simulink model "mechatronic_system_ss"  (R2023b)
settings: Solver=ode1  StartTime=0.0  StopTime=inf  FixedStep=time_step  RelTol=1e-3  EnableMultiTasking=on
model workspace (MAT data in the model file):
  A_ss = [0  1  0  0  0  0; 0  -10.6382978723  0  -2.12765957447  0  0; 0  0  0  1  0  0; 0  8.33333333333  -16666.6666667  -184.166666667  166666.666667  0; 0  0  0  0  0  1; 0  0  1000  0  -10000  -1.5]
  B_ss = [0  0  0  0  0  0; 0  1  0  0  0  0; 0  0  0  0  0  0; 0  0  0  0  0  0; 0  0  0  0  0  0; 0  0  0  0  0  1]
  C_ss = [1  0  0  0  0  0; 0  1  0  0  0  0; 0  0  1  0  0  0; 0  0  0  1  0  0; 0  0  0  0  1  0; 0  0  0  0  0  1]
  Cm = 0.1
  D_ss = [0  0  0  0  0  0; 0  0  0  0  0  0; 0  0  0  0  0  0; 0  0  0  0  0  0; 0  0  0  0  0  0; 0  0  0  0  0  0]
  J_shaft = 0.012
  Ja = 0.001
  La = 0.047
  Ra = 0.5
  b_shaft = 2.21
  b_spring = 3
  ba = 0.01
  g = 9.81
  k_spring = 20000
  lower_limit = 0
  m = 2
  r_shaft = 0.1
  time_step = 0.002
  upper_limit = 5
libraries: simulink x1
settings Model: Creator=danie  LastModifiedBy=danie
settings SolverCC: AutoInsertRateTranBlk=on  InsertRTBMode=Always
settings OptimizationCC: DefaultParameterBehavior=Inlined  EnhancedBackFolding=on  PassReuseOutputArgsAs=Individual arguments  ZeroExternalMemoryAtStartup=off  ZeroInternalMemoryAtStartup=off  OptimizeBlockOrder=speed  DifferentSizesBufferReuse=on  OptimizationCustomize=off  EfficientTunableParamExpr=on
settings DebuggingCC: ParameterTunabilityLossMsg=error
settings HardwareCC: ProdBitPerLong=64  ProdHWDeviceType=Intel->x86-64 (Linux 64)
settings SFSimCC: MATLABDynamicMemAlloc=off
settings RTWCC: Description=Embedded Coder  SystemTargetFile=ert.tlc  GenCodeOnly=on  PackageGeneratedCodeAndArtifacts=on  TemplateMakefile=ert_default_tmf
settings CodeAppCC: ForceParamTrailComments=on  IgnoreCustomStorageClasses=off  OperatorAnnotations=on  SimulinkDataObjDesc=on  SFDataObjDesc=on  InsertBlockDesc=on
settings ERTTargetCC: TargetLangStandard=C99 (ISO)  GenerateSampleERTMain=on  SupportContinuousTime=on  InlinedParameterPlacement=NonHierarchical  ERTCustomFileTemplate=example_file_process.tlc

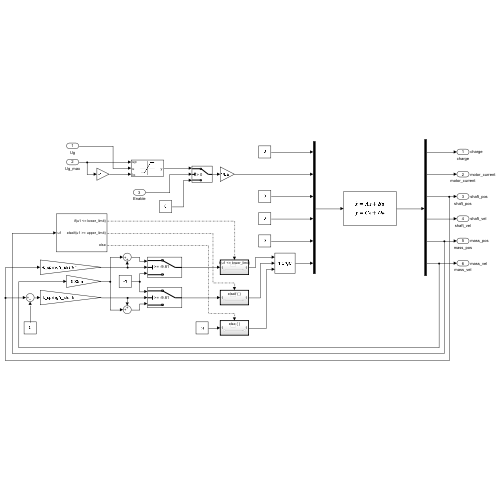
[thumbnail: Simulink's stored preview of the top-level diagram]
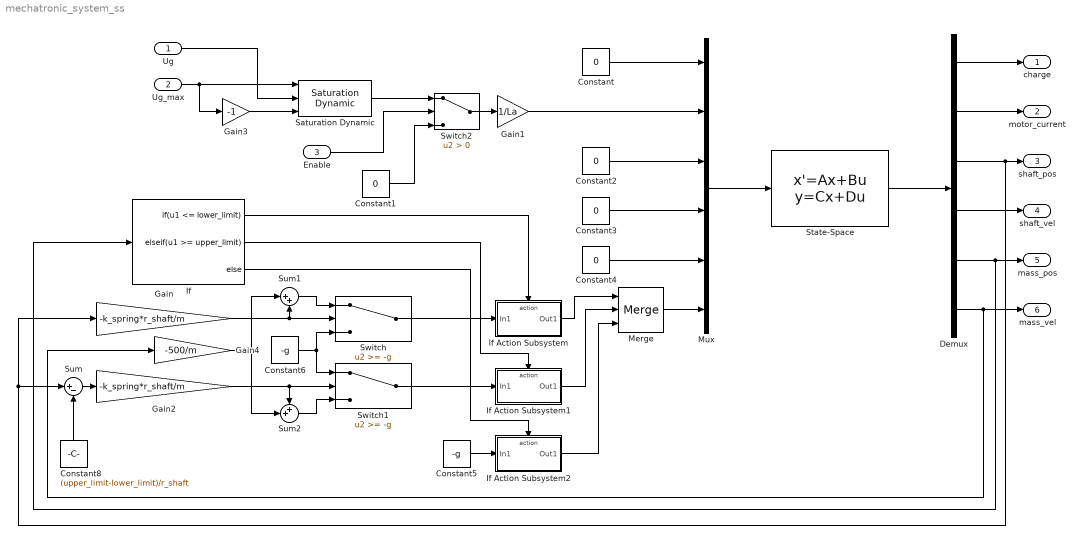
== system mechatronic_system_ss ==
  Ug : Inport
  Ug_max : Inport  Port=2
  Enable : Inport  Port=3
  Constant{,1..4} (5 alike) : Constant  Value=0
  Constant5 : Constant  Value=-g
  Constant6 : Constant  Value=-g
  Constant8 : Constant  Value=(upper_limit-lower_limit)/r_shaft
  Demux : Demux  Outputs=6
  Gain : Gain  Gain=-k_spring*r_shaft/m
  Gain1 : Gain  Gain=1/La
  Gain2 : Gain  Gain=-k_spring*r_shaft/m
  Gain3 : Gain  Gain=-1
  Gain4 : Gain  Gain=-500/m
  If : If  IfExpression=u1 <= lower_limit  ElseIfExpressions=u1 >= upper_limit
  If Action Subsystem : Subsystem  TreatAsAtomicUnit=on
  If Action Subsystem1 : Subsystem  TreatAsAtomicUnit=on
  If Action Subsystem2 : Subsystem  TreatAsAtomicUnit=on
  Merge : Merge  Inputs=3
  Mux : Mux  Inputs=6
  Saturation Dynamic : simulink/Discontinuities/Saturation Dynamic  OutMin=[]  OutMax=[]  OutDataTypeStr=Inherit: Same as second input  OutDataType=fixdt(1, 16)  OutScaling=2^-10  DoSatur=off
  State-Space : StateSpace  A=A_ss  B=B_ss  C=C_ss  D=D_ss  InitialCondition=0
  Sum : Sum  Inputs=|+-
  Sum1 : Sum  Inputs=|++
  Sum2 : Sum  Inputs=++|
  Switch : Switch  Threshold=-g  SaturateOnIntegerOverflow=off  InputSameDT=off
  Switch1 : Switch  Threshold=-g  SaturateOnIntegerOverflow=off  InputSameDT=off
  Switch2 : Switch  Criteria=u2 > Threshold  SaturateOnIntegerOverflow=off  InputSameDT=off
  charge : Outport  SignalName=charge
  motor_current : Outport  Port=2  SignalName=motor_current
  shaft_pos : Outport  Port=3  SignalName=shaft_pos
  shaft_vel : Outport  Port=4  SignalName=shaft_vel
  mass_pos : Outport  Port=5  SignalName=mass_pos
  mass_vel : Outport  Port=6  SignalName=mass_vel
  wires:
  Mux/1 -> State-Space/1
  State-Space/1 -> Demux/1
  Constant/1 -> Mux/1
  Gain1/1 -> Mux/2
  Constant2/1 -> Mux/3
  Constant3/1 -> Mux/4
  Constant4/1 -> Mux/5
  Demux/1 -> charge/1
  Demux/2 -> motor_current/1
  Demux/4 -> shaft_vel/1
  Demux/3 -> shaft_pos/1, Sum/1, Gain/1
  Demux/5 -> mass_pos/1, If/1
  Demux/6 -> Gain4/1, mass_vel/1
  If/1 -> If Action Subsystem/Action
  If/2 -> If Action Subsystem1/Action
  If/3 -> If Action Subsystem2/Action
  Merge/1 -> Mux/6
  If Action Subsystem/1(Out1) -> Merge/1
  If Action Subsystem1/1(Out1) -> Merge/2
  If Action Subsystem2/1(Out1) -> Merge/3
  Switch/1 -> If Action Subsystem/1(In1)
  Switch1/1 -> If Action Subsystem1/1(In1)
  Gain/1 -> Sum1/2, Switch/2
  Constant5/1 -> If Action Subsystem2/1(In1)
  Constant6/1 -> Switch1/1, Switch/3
  Sum/1 -> Gain2/1
  Gain2/1 -> Sum2/1, Switch1/2
  Constant8/1 -> Sum/2
  Gain3/1 -> Saturation Dynamic/3
  Ug/1 -> Saturation Dynamic/2
  Ug_max/1 -> Gain3/1, Saturation Dynamic/1
  Switch2/1 -> Gain1/1
  Saturation Dynamic/1 -> Switch2/1
  Constant1/1 -> Switch2/3
  Enable/1 -> Switch2/2
  Sum1/1 -> Switch/1
  Sum2/1 -> Switch1/3
  Gain4/1 -> Sum1/1, Sum2/2

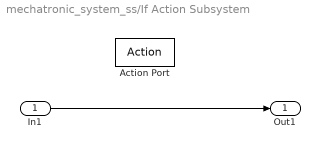
== system mechatronic_system_ss/If Action Subsystem ==
  In1 : Inport
  Action Port : ActionPort  ActionPortLabel=if(u1 <= lower_limit)
  Out1 : Outport
  wires:
  In1/1 -> Out1/1

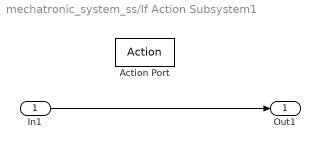
== system mechatronic_system_ss/If Action Subsystem1 ==
  In1 : Inport
  Action Port : ActionPort  ActionPortLabel=elseif(u1 >= upper_limit)
  Out1 : Outport
  wires:
  In1/1 -> Out1/1

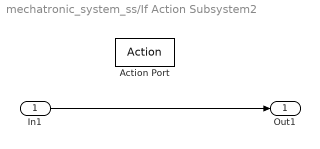
== system mechatronic_system_ss/If Action Subsystem2 ==
  In1 : Inport
  Action Port : ActionPort  ActionPortLabel=else
  Out1 : Outport
  wires:
  In1/1 -> Out1/1
